simulink model "Glide_slope_modelv3"  (R2020a)
settings: Solver=VariableStepAuto  StartTime=0.0  StopTime=160  RelTol=1e-3
undefined symbols (not defined in the file or in its folder): med_AA, med_BB, med_CC, med_DD, trim_control_lo, trim_thrust_lo
libraries: simulink_extras x1, simulink x1
settings Model: Creator=mathi  LastModifiedBy=Nico

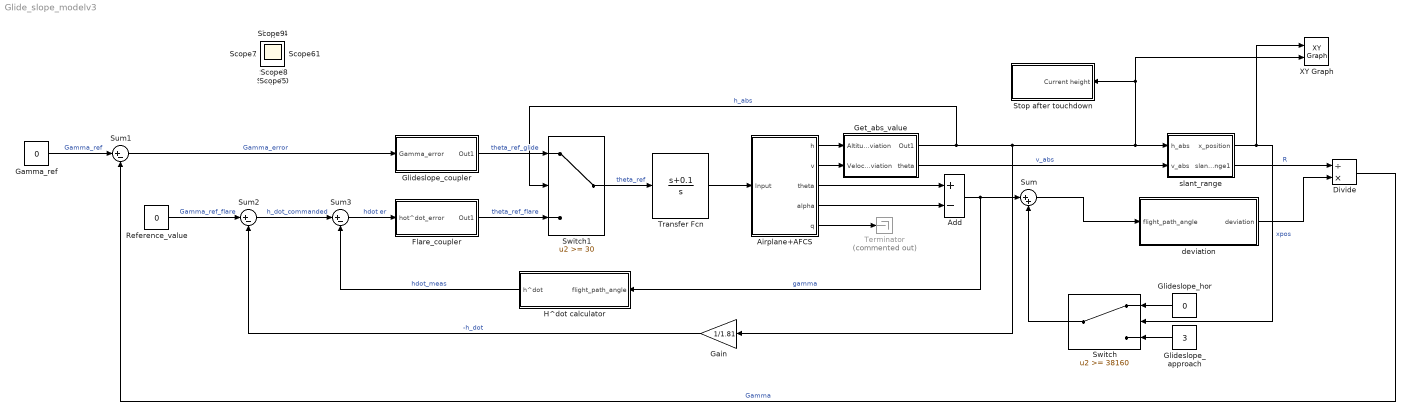
== system Glide_slope_modelv3 ==
  Add : Sum  Inputs=+-
  Airplane+AFCS : Subsystem
  Divide : Product  Inputs=/*
  Flare_coupler : Subsystem
  Gain : Gain  Gain=1/1.81
  Gamma_ref : Constant  Value=0
  Get_abs_value : Subsystem
  Glideslope_approach : Constant  Value=3
  Glideslope_coupler : Subsystem
  Glideslope_hor : Constant  Value=0
  H^dot calculator : Subsystem
  Reference_value : Constant  Value=0
  Stop after touchdown : Subsystem
  Sum : Sum  Inputs=|++
  Sum1 : Sum  Inputs=|+-
  Sum2 : Sum  Inputs=|+-
  Sum3 : Sum  Inputs=|+-
  Switch : Switch  Threshold=38160
  Switch1 : Switch  Threshold=30
  Terminator : Terminator  Commented=on
  Transfer Fcn : TransferFcn  Numerator=[1 0.1]  Denominator=[1 0]
  XY Graph : simulink/Sinks/XY Graph  xmin=-800  xmax=42000  ymin=-1  ymax=2000  st=-1
  deviation : Subsystem
  slant_range : Subsystem
  Scope{,1..11} (12 alike) : Scope
  wires:
  Add/1 -> Sum/1, H^dot calculator/1(flight_path_angle)  "gamma"
  Sum1/1 -> Glideslope_coupler/1(Gamma_error)  "Gamma_error"
  Gamma_ref/1 -> Sum1/1  "Gamma_ref"
  Airplane+AFCS/4(alpha) -> Add/2
  Get_abs_value/2(theta) -> slant_range/2(v_abs)  "v_abs"
  Divide/1 -> Sum1/2  "Gamma"
  Airplane+AFCS/3(theta) -> Add/1
  Airplane+AFCS/2(v) -> Get_abs_value/2(Velocity_deviation)
  Airplane+AFCS/1(h) -> Get_abs_value/1(Altitude_deviation)
  Airplane+AFCS/5(q) -> Terminator/1
  Get_abs_value/1(Out1) -> Gain/1, XY Graph/2, Stop after touchdown/1(Current height), slant_range/1(h_abs), Switch1/2  "h_abs"
  Sum/1 -> deviation/1(flight_path_angle)
  deviation/1(deviation) -> Divide/2
  slant_range/2(slant_range1) -> Divide/1  "R"
  slant_range/1(x_position) -> XY Graph/1, Switch/2  "xpos"
  Glideslope_approach/1 -> Switch/3
  Glideslope_hor/1 -> Switch/1
  Switch/1 -> Sum/2
  Glideslope_coupler/1(Out1) -> Switch1/1  "theta_ref_glide"
  Flare_coupler/1(Out1) -> Switch1/3  "theta_ref_flare"
  Reference_value/1 -> Sum2/1  "Gamma_ref_flare"
  Sum3/1 -> Flare_coupler/1(hot^dot_error)  "hdot er"
  Sum2/1 -> Sum3/1  "h_dot_commanded"
  Gain/1 -> Sum2/2  "-h_dot"
  H^dot calculator/1(h^dot) -> Sum3/2  "hdot_meas"
  Switch1/1 -> Transfer Fcn/1  "theta_ref"
  Transfer Fcn/1 -> Airplane+AFCS/1(Input)

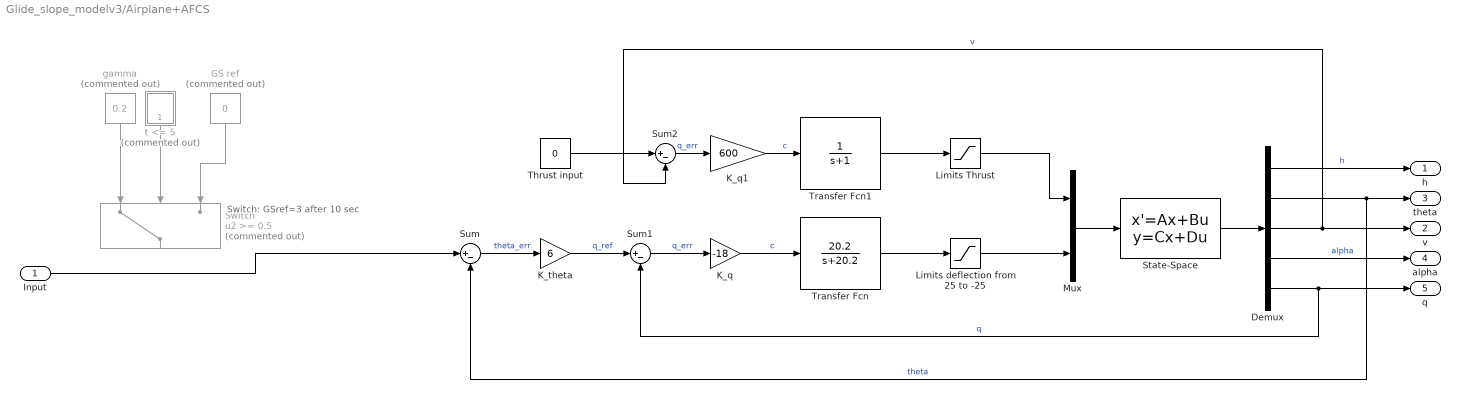
== system Glide_slope_modelv3/Airplane+AFCS ==
  note: Switch:
      | GSref=3 after 10 sec
  Input : Inport
  Demux : Demux  Outputs=5
  GS ref : Constant  Commented=on  Value=0
  K_q : Gain  Gain=-18
  K_q1 : Gain  Gain=600
  K_theta : Gain  Gain=6
  Limits Thrust : Saturate  UpperLimit=19000-trim_thrust_lo  LowerLimit=1000-trim_thrust_lo
  Limits deflection from 25 to -25 : Saturate  UpperLimit=25-trim_control_lo(1)  LowerLimit=-25-trim_control_lo(1)
  Mux : Mux  Inputs=2
  State-Space : StateSpace  A=med_AA  B=med_BB  C=med_CC  D=med_DD  InitialCondition=0
  Sum : Sum  Inputs=|+-
  Sum1 : Sum  Inputs=|+-
  Sum2 : Sum  Inputs=|+-
  Switch : Switch  Commented=on  Threshold=0.5
  Thrust input : Constant  Value=0
  Transfer Fcn : TransferFcn  Numerator=[0 20.2]  Denominator=[1 20.2]
  Transfer Fcn1 : TransferFcn  Numerator=[0 1]  Denominator=[1 1]
  gamma : Constant  Commented=on  Value=0.2
  t <= 5 : Subsystem  Commented=on
  h : Outport
  v : Outport  Port=2
  theta : Outport  Port=3
  alpha : Outport  Port=4
  q : Outport  Port=5
  wires:
  Sum/1 -> K_theta/1  "theta_err"
  K_theta/1 -> Sum1/1  "q_ref"
  Sum1/1 -> K_q/1  "q_err"
  K_q/1 -> Transfer Fcn/1  "c"
  Transfer Fcn/1 -> Limits deflection from 25 to -25/1
  Limits deflection from 25 to -25/1 -> Mux/2
  Mux/1 -> State-Space/1
  Demux/2 -> theta/1, Sum/2  "theta"
  State-Space/1 -> Demux/1
  Demux/5 -> Sum1/2, q/1  "q"
  Demux/4 -> alpha/1  "alpha"
  Demux/3 -> Sum2/2, v/1  "v"
  Demux/1 -> h/1  "h"
  GS ref/1 -> Switch/3
  gamma/1 -> Switch/1
  t <= 5/1(t < =10) -> Switch/2
  Input/1 -> Sum/1
  Thrust input/1 -> Sum2/1
  Sum2/1 -> K_q1/1  "q_err"
  Transfer Fcn1/1 -> Limits Thrust/1
  Limits Thrust/1 -> Mux/1
  K_q1/1 -> Transfer Fcn1/1  "c"

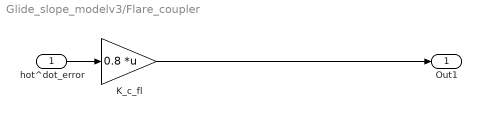
== system Glide_slope_modelv3/Flare_coupler ==
  hot^dot_error : Inport
  K_c_fl : Gain  Gain=0.8  Multiplication=Matrix(K*u)
  Out1 : Outport
  wires:
  hot^dot_error/1 -> K_c_fl/1
  K_c_fl/1 -> Out1/1

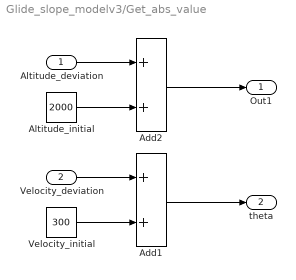
== system Glide_slope_modelv3/Get_abs_value ==
  Altitude_deviation : Inport
  Velocity_deviation : Inport  Port=2
  Add1 : Sum
  Add2 : Sum
  Altitude_initial : Constant  Value=2000
  Velocity_initial : Constant  Value=300
  Out1 : Outport
  theta : Outport  Port=2
  wires:
  Velocity_deviation/1 -> Add1/1
  Velocity_initial/1 -> Add1/2
  Add1/1 -> theta/1
  Altitude_deviation/1 -> Add2/1
  Altitude_initial/1 -> Add2/2
  Add2/1 -> Out1/1

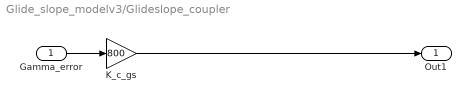
== system Glide_slope_modelv3/Glideslope_coupler ==
  Gamma_error : Inport
  K_c_gs : Gain  Gain=800
  Out1 : Outport
  wires:
  K_c_gs/1 -> Out1/1
  Gamma_error/1 -> K_c_gs/1

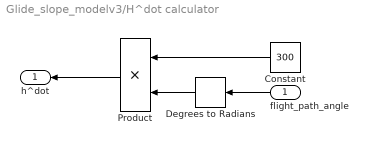
== system Glide_slope_modelv3/H^dot calculator ==
  flight_path_angle : Inport
  Constant : Constant  Value=300
  Degrees to Radians : simulink_extras/Transformations/Degrees to Radians
  Product : Product
  h^dot : Outport
  wires:
  Constant/1 -> Product/1
  Product/1 -> h^dot/1
  flight_path_angle/1 -> Degrees to Radians/1
  Degrees to Radians/1 -> Product/2

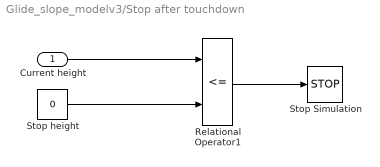
== system Glide_slope_modelv3/Stop after touchdown ==
  Current height : Inport
  Relational Operator1 : RelationalOperator  Operator=<=  OutDataTypeStr=boolean  RndMeth=Simplest
  Stop Simulation : Stop
  Stop height : Constant  Value=0
  wires:
  Current height/1 -> Relational Operator1/1
  Relational Operator1/1 -> Stop Simulation/1
  Stop height/1 -> Relational Operator1/2

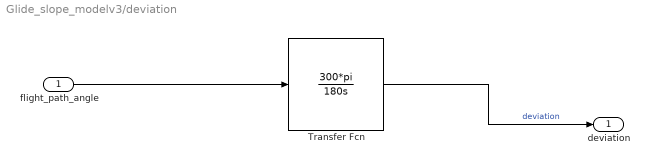
== system Glide_slope_modelv3/deviation ==
  flight_path_angle : Inport
  Transfer Fcn : TransferFcn  Numerator=300*pi  Denominator=[180 0]
  deviation : Outport
  wires:
  flight_path_angle/1 -> Transfer Fcn/1
  Transfer Fcn/1 -> deviation/1  "deviation"

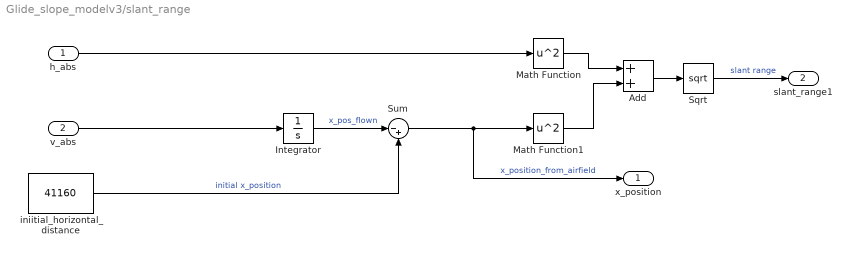
== system Glide_slope_modelv3/slant_range ==
  h_abs : Inport
  v_abs : Inport  Port=2
  Add : Sum
  Integrator : Integrator
  Math Function : Math  Operator=square  SaturateOnIntegerOverflow=on
  Math Function1 : Math  Operator=square  SaturateOnIntegerOverflow=on
  Sqrt : Sqrt  SaturateOnIntegerOverflow=on
  Sum : Sum  Inputs=|-+
  iniitial_horizontal_distance : Constant  Value=41160
  x_position : Outport
  slant_range1 : Outport  Port=2
  wires:
  h_abs/1 -> Math Function/1
  v_abs/1 -> Integrator/1
  iniitial_horizontal_distance/1 -> Sum/2  "initial x_position"
  Integrator/1 -> Sum/1  "x_pos_flown"
  Sum/1 -> x_position/1, Math Function1/1  "x_position_from_airfield"
  Math Function/1 -> Add/1
  Math Function1/1 -> Add/2
  Add/1 -> Sqrt/1
  Sqrt/1 -> slant_range1/1  "slant range"

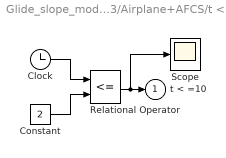
== system Glide_slope_modelv3/Airplane+AFCS/t <= 5 ==
  Clock : Clock
      settings: Decimation=100
  Constant : Constant  Value=2
  Relational Operator : RelationalOperator  Operator=<=  RndMeth=Nearest  InputSameDT=on
  Scope : Scope
  t < =10 : Outport  InitialOutput=0  VectorParamsAs1DForOutWhenUnconnected=off
  wires:
  Constant/1 -> Relational Operator/2
  Clock/1 -> Relational Operator/1
  Relational Operator/1 -> Scope/1, t < =10/1
